simulink model "Part1_e_simu"  (R2018b)
settings: Solver=VariableStepAuto  StartTime=0.0  StopTime=200  RelTol=1e-3
values from neighbouring files (symbols this model uses):
  b = 62    [Part1_d.m]    (also in Part1_e.m)
  Fgrav = m * g *sind(theta)    [Part1_e.m]
  Fwheels_max = 4 * Tmax / r    (= 24416.6666667)    [Part1_d.m]    (also in Part1_e.m)
  Fwheels_ss = 4 * Tss / r    (= 1663.33333333)    [Part1_d.m]    (also in Part1_e.m)
  m = 2110    [Part1_d.m]    (also in Part1_e.m)
settings Model: Creator=Nick Carcione  LastModifiedBy=Nick Carcione

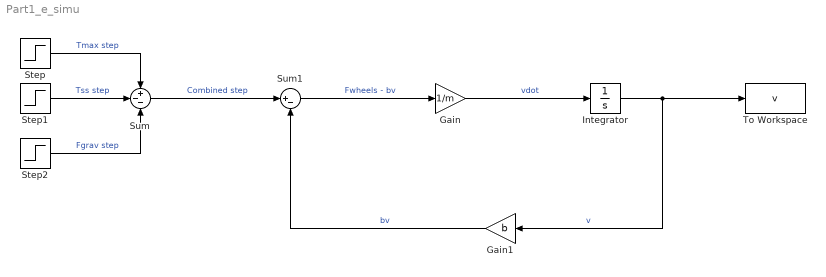
== system Part1_e_simu ==
  Gain : Gain  Gain=1/m
  Gain1 : Gain  Gain=b
  Integrator : Integrator
  Step : Step  Time=0  After=Fwheels_max  SampleTime=0
  Step1 : Step  Time=2.4  After=Fwheels_max - Fwheels_ss  SampleTime=0
  Step2 : Step  Time=10  After=Fgrav  SampleTime=0
  Sum : Sum  Inputs=+--
  Sum1 : Sum  Inputs=|+-
  To Workspace : ToWorkspace  VariableName=v  SaveFormat=Timeseries  SampleTime=-1
  wires:
  Step/1 -> Sum/1  "Tmax step"
  Gain/1 -> Integrator/1  "vdot"
  Gain1/1 -> Sum1/2  "bv"
  Step1/1 -> Sum/2  "Tss step"
  Sum1/1 -> Gain/1  "Fwheels - bv"
  Sum/1 -> Sum1/1  "Combined step"
  Integrator/1 -> Gain1/1, To Workspace/1  "v"
  Step2/1 -> Sum/3  "Fgrav step"
